simulink model "pom1wg_kot_2010"  (Simulink 7.6)
settings: Solver=ode45  SolverMode=SingleTasking  StartTime=0.0  StopTime=3000  MaxStep=1  RelTol=1e-3  AbsTol=1e-6
undefined symbols (not defined in the file): cpw, Cvg, Cvk, Cvws, czas_skok, dFg, dQk, dQt, dTzew, Fg0, Kcg, Kcw, Qk0, Qt0, Tgp0, Tkz0, To, Twew0, Tzew0
settings Model: Creator=ac  LastModifiedBy=ac  ExtModeTrigMode=oneshot  ExtModeArmWhenConnect=off
settings DataIOCC: LimitDataPoints=off
settings OptimizationCC: BlockReduction=off  BooleanDataType=off
settings DebuggingCC: SaveWithParameterizedLinksMsg=none  SignalResolutionControl=TryResolveAllWithWarning  SolverPrmCheckMsg=none  MultiTaskDSMMsg=warning  MultiTaskCondExecSysMsg=none  StrictBusMsg=None
settings HardwareCC: TargetUnknown=on
settings RTWCC: IncludeERTFirstTime=on

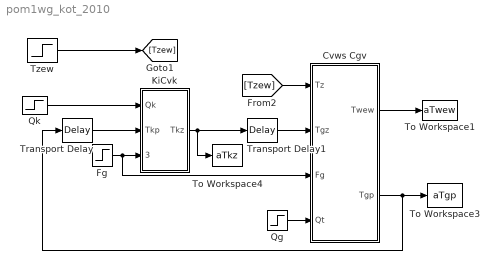
== system pom1wg_kot_2010 ==
  Cvws Cgv : Subsystem
  Fg : Step  Time=czas_skok  Before=Fg0  After=Fg0+dFg  SampleTime=0
  KiCvk : Subsystem  mask{cpw=cpw, Cvk=Cvk, Tkz0=Tkz0}
  Qg : Step  Time=czas_skok  Before=Qt0  After=Qt0+dQt  SampleTime=0
  Qk : Step  Time=czas_skok  Before=Qk0  After=Qk0+dQk  SampleTime=0
  To Workspace1 : ToWorkspace  VariableName=aTwew  SampleTime=-1  SaveFormat=Array
  To Workspace3 : ToWorkspace  VariableName=aTgp  SampleTime=-1  SaveFormat=Array
  To Workspace4 : ToWorkspace  VariableName=aTkz  SampleTime=-1  SaveFormat=Array
  Transport Delay : TransportDelay  DelayTime=To  InitialOutput=Tgp0
  Transport Delay1 : TransportDelay  DelayTime=To  InitialOutput=Tkz0
  Tzew : Step  Time=czas_skok  Before=Tzew0  After=Tzew0+dTzew  SampleTime=0
  wires:
  Fg/1 -> KiCvk/3(Fgm), Cvws Cgv/3(Fg)
  Transport Delay/1 -> KiCvk/2(Tkp)
  Qg/1 -> Cvws Cgv/4(Qt)
  Cvws Cgv/1(Twew) -> To Workspace1/1
  Cvws Cgv/2(Tgp) -> To Workspace3/1, Transport Delay/1
  Transport Delay1/1 -> Cvws Cgv/2(Tgz)
  [Tzew] -> Cvws Cgv/1(Tz)
  KiCvk/1(Tkz) -> Transport Delay1/1, To Workspace4/1
  Qk/1 -> KiCvk/1(Qk)
  Tzew/1 -> [Tzew]

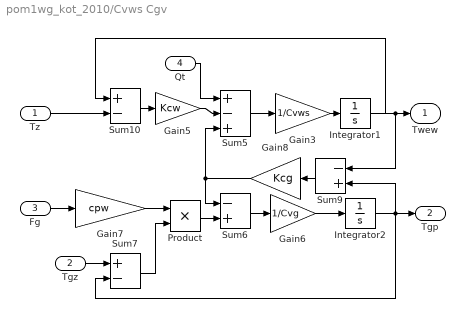
== system pom1wg_kot_2010/Cvws Cgv ==
  Tz : Inport
  Tgz : Inport  Port=2
  Fg : Inport  Port=3
  Qt : Inport  Port=4
  Gain3 : Gain  Gain=1/Cvws  SaturateOnIntegerOverflow=on  OutDataTypeStr=Inherit: Same as input  ParamDataTypeStr=Inherit: Same as input
  Gain5 : Gain  Gain=Kcw  SaturateOnIntegerOverflow=on  OutDataTypeStr=Inherit: Same as input  ParamDataTypeStr=Inherit: Same as input
  Gain6 : Gain  Gain=1/Cvg  SaturateOnIntegerOverflow=on  OutDataTypeStr=Inherit: Same as input  ParamDataTypeStr=Inherit: Same as input
  Gain7 : Gain  Gain=cpw  SaturateOnIntegerOverflow=on  OutDataTypeStr=Inherit: Same as input  ParamDataTypeStr=Inherit: Same as input
  Gain8 : Gain  Gain=Kcg  SaturateOnIntegerOverflow=on  OutDataTypeStr=Inherit: Same as input  ParamDataTypeStr=Inherit: Same as input
  Integrator1 : Integrator  InitialCondition=Twew0
  Integrator2 : Integrator  InitialCondition=Tgp0
  Product : Product  SaturateOnIntegerOverflow=on  RndMeth=Zero  InputSameDT=on  OutDataTypeStr=Inherit: Same as first input
  Sum10 : Sum  Inputs=+-  SaturateOnIntegerOverflow=on  InputSameDT=on  OutDataTypeStr=Inherit: Same as first input
  Sum5 : Sum  Inputs=+-+  SaturateOnIntegerOverflow=on  InputSameDT=on  OutDataTypeStr=Inherit: Same as first input
  Sum6 : Sum  Inputs=-+  SaturateOnIntegerOverflow=on  InputSameDT=on  OutDataTypeStr=Inherit: Same as first input
  Sum7 : Sum  Inputs=+-  SaturateOnIntegerOverflow=on  InputSameDT=on  OutDataTypeStr=Inherit: Same as first input
  Sum9 : Sum  Inputs=-+  SaturateOnIntegerOverflow=on  InputSameDT=on  OutDataTypeStr=Inherit: Same as first input
  Twew : Outport
  Tgp : Outport  Port=2
  wires:
  Sum5/1 -> Gain3/1
  Sum6/1 -> Gain6/1
  Gain7/1 -> Product/1
  Sum7/1 -> Product/2
  Product/1 -> Sum6/2
  Gain6/1 -> Integrator2/1
  Integrator2/1 -> Sum7/2, Sum9/2, Tgp/1
  Sum9/1 -> Gain8/1
  Gain3/1 -> Integrator1/1
  Integrator1/1 -> Sum9/1, Sum10/1, Twew/1
  Sum10/1 -> Gain5/1
  Gain8/1 -> Sum6/1, Sum5/3
  Gain5/1 -> Sum5/2
  Qt/1 -> Sum5/1
  Fg/1 -> Gain7/1
  Tgz/1 -> Sum7/1
  Tz/1 -> Sum10/2

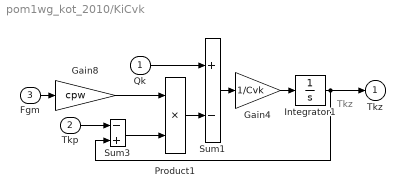
== system pom1wg_kot_2010/KiCvk ==
  note: Tkz
  Qk : Inport
  Tkp : Inport  Port=2
  Fgm : Inport  Port=3
  Gain4 : Gain  Gain=1/Cvk  SaturateOnIntegerOverflow=on  OutDataTypeStr=Inherit: Same as input  ParamDataTypeStr=Inherit: Same as input
  Gain8 : Gain  Gain=cpw  SaturateOnIntegerOverflow=on  OutDataTypeStr=Inherit: Same as input  ParamDataTypeStr=Inherit: Same as input
  Integrator1 : Integrator  InitialCondition=Tkz0
  Product1 : Product  Inputs=**  SaturateOnIntegerOverflow=on  RndMeth=Zero  InputSameDT=on  OutDataTypeStr=Inherit: Same as first input
  Sum1 : Sum  Inputs=+-  SaturateOnIntegerOverflow=on  InputSameDT=on  OutDataTypeStr=Inherit: Same as first input
  Sum3 : Sum  Inputs=-+  SaturateOnIntegerOverflow=on  InputSameDT=on  OutDataTypeStr=Inherit: Same as first input
  Tkz : Outport
  wires:
  Tkp/1 -> Sum3/1
  Integrator1/1 -> Sum3/2, Tkz/1
  Product1/1 -> Sum1/2
  Sum1/1 -> Gain4/1
  Gain4/1 -> Integrator1/1
  Qk/1 -> Sum1/1
  Gain8/1 -> Product1/1
  Sum3/1 -> Product1/2
  Fgm/1 -> Gain8/1
